simulink model "PilotModelUnitTest"  (R2018b)
settings: Solver=VariableStepAuto  StartTime=0.0  StopTime=100  RelTol=1e-3
values from neighbouring files (symbols this model uses):
  enableHorzMan = 1    [unitTest_PilotModel.m]
  enableVertMan = 0    [unitTest_PilotModel.m]
undefined symbols (not defined in the file or in its folder): ac2dyn_alt0_ft, ac2dyn_con, ac2dyn_lat0_rad, ac2dyn_lon0_rad, daaLogic_turnRate_dps, daaLogic_vertRate_fpm, ddh_ftps2, dh_ftps, dv_ftps2, e_ft, Edot_ftps, h_ft, hdot_ftps, latLonAltState, n_ft, Ndot_ftps, p_radps, phi_rad, phidot_radps, psi_rad, psidot_radps, q_radps, r_radps, theta_rad, thetadot_radps, uasPilot_altitudeK, uasPilot_altitudeOffset, uasPilot_altitudeTheta, uasPilot_coordDelayK, uasPilot_coordDelayMin, uasPilot_coordDelayTheta, uasPilot_desiredTurnRate_dps, uasPilot_desiredVertRate_ftpm, uasPilot_deterministicMode, uasPilot_dt_s, uasPilot_executionDelayMin, uasPilot_executionDelayMu, uasPilot_initialDelayMin, uasPilot_initialDelayMu, uasPilot_maxRelativeHdg, uasPilot_meanUpdateTimes, uasPilot_mentalFilter_climbThresh_fps, uasPilot_mentalFilter_numSamp, uasPilot_mentalFilter_turnThresh_rad, uasPilot_minUpdateTimes, uasPilot_operatorEnabled, uasPilot_probDescend, uasPilot_probFollowMinDev, uasPilot_probLeftTurn, uasPilot_probTurn, uasPilot_reducedClimbAlt_ft, uasPilot_reducedTurnAngle_deg, uasPilot_seedChoose, uasPilot_seedCoordDelay, uasPilot_seedExecutionDelay, uasPilot_seedInitialDelay, uasPilot_seedTurn, uasPilot_seedUpdate, uasPilot_seedVertical, uasPilot_triggerLevel ... (+8)
libraries: simulink x17, NullAircraftEstimateBus x1, uas_pilot_model_r6 x1
(part 1 of 2)
settings Model: Creator=PE29732  LastModifiedBy=BI28030

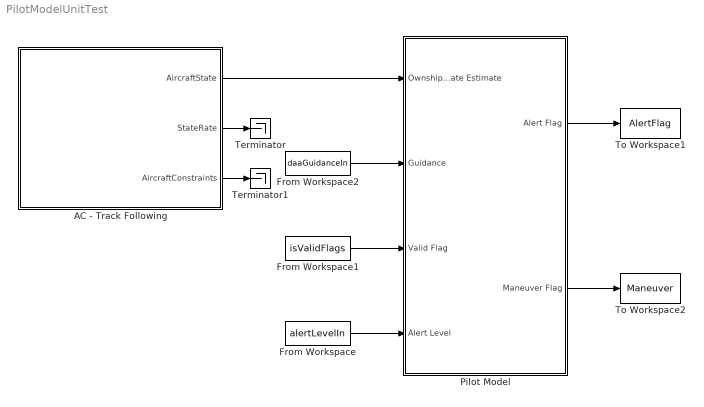
== system PilotModelUnitTest ==
  AC - Track Following : Subsystem  mask(Basic Aircraft Dynamic Model){ts_dynamics=0.1, lat0_rad=ac2dyn_lat0_rad, lon0_rad=ac2dyn_lon0_rad, alt_ft=ac2dyn_alt0_ft, v_ftps_max=ac2dyn_con.maxAirspeed_ftps, v_ftps_min=ac2dyn_con.minAirspeed_ftps, dv_ftpss_max=ac2dyn_con.maxAcceleration_ftpss, dv_ftpss_min=ac2dyn_con.minAcceleration_ftpss, dh_ftps_max=ac2dyn_con.maxVerticalRate_ftps, dh_ftps_min=ac2dyn_con.minVerticalRate_ftps, q_radps_max=ac2dyn_con.maxPitchRate_radps, phi_rad_max=ac2dyn_con.maxBankAngle_rad, dphi_radps_max=ac2dyn_con.maxRollRate_radps, r_radps_max=ac2dyn_con.maxYawRate_radps, pNUM=ac2dyn_con.dynamicsNumeratorRollRate, pDEN=ac2dyn_con.dynamicsDenominatorRollRate, hNUM=ac2dyn_con.dynamicsNumeratorVerticalRate, hDEN=ac2dyn_con.dynamicsDenominatorVerticalRate, rNUM=ac2dyn_con.dynamicsNumeratorYawRate, rDEN=ac2dyn_con.dynamicsDenominatorYawRate}
      mask prompts: ts_dynamics "Dynamics update parameter"; lat0_rad "Latitude of ENU origin (rad)"; lon0_rad "Longitude of ENU origin (rad)"; alt_ft "Height of ENU origin (ft)"; v_ftps_max "Maximum airspeed (ft/s)"; v_ftps_min "Minimum airspeed (ft/s)"; dv_ftpss_max "Maximum acceleration (ft/s/s)"; dv_ftpss_min "Miniimum acceleration (ft/s/s)"; dh_ftps_max "Maximum vertical rate (ft/s)"; dh_ftps_min "Minimum vertical rate (ft/s)"; q_radps_max "Maximum pitch rate (rad/s)"; phi_rad_max "Maximum bank angle (rad)"; dphi_radps_max "Maximum roll rate (rad/s)"; r_radps_max "Maximum yaw rate (rad/s)"; pNUM "Roll rate discrete dynamics numerator (2x1)"; pDEN "Roll rate discrete dynamics denominator (1x1)"; hNUM "Vertical rate discrete dynamics numerator (2x1)"; hDEN "Vertical rate discrete dynamics denominator (1x1)"; rNUM "Yaw rate discrete dynamics numerator (2x1)"; rDEN "Yaw rate discrete dynamics denominator (1x1)"
      mask help:
      | Propagates the aircraft dynamics using 6DOF equations of motion.
      |
      | The class Simple6DOF can be used to programmatically set the parameters of Basic Aircraft Dynamcis blocks.
      mask Help:
      | Propagates the aircraft dynamics using 6DOF equations of motion.
      | 
      | The class Simple6DOF can be used to programmatically set the parameters of Basic Aircraft Dynamcis blocks.
      mask DialogControl ParameterTabVar0 Prompt: Main
      mask DialogControl ParameterTabVar01 Prompt: Constraints
  From Workspace : FromWorkspace  VariableName=alertLevelIn  SampleTime=0
  From Workspace1 : FromWorkspace  VariableName=isValidFlags  SampleTime=0
  From Workspace2 : FromWorkspace  VariableName=daaGuidanceIn  SampleTime=0
  Pilot Model : Subsystem  mask(Heuristic Operator Model){dt=uasPilot_dt_s, operator_enabled=uasPilot_operatorEnabled, deterministicMode=uasPilot_deterministicMode, trigger_level=uasPilot_triggerLevel, mean_initial_delay=uasPilot_initialDelayMu, min_initial_delay=uasPilot_initialDelayMin, coord_delay_k=uasPilot_coordDelayK, coord_delay_theta=uasPilot_coordDelayTheta, coord_delay_min=uasPilot_coordDelayMin, mean_exec_delay=uasPilot_executionDelayMu, min_exec_delay=uasPilot_executionDelayMin, min_upd_times=uasPilot_minUpdateTimes, mean_upd_times=uasPilot_meanUpdateTimes, rng_seed_initial=uasPilot_seedInitialDelay, rng_seed_coord=uasPilot_seedCoordDelay, rng_seed_execution=uasPilot_seedExecutionDelay, rng_seed_update=uasPilot_seedUpdate, prob_follow_min=uasPilot_probFollowMinDev, prob_turn_left=uasPilot_probLeftTurn, prob_descend=uasPilot_probDescend, prob_turn=uasPilot_probTurn, max_hdg_diff=uasPilot_maxRelativeHdg, turn_k=uasPilot_turnK, turn_theta=uasPilot_turnTheta, turn_offset=uasPilot_turnOffset, alt_k=uasPilot_altitudeK, alt_theta=uasPilot_altitudeTheta, alt_offset=uasPilot_altitudeOffset, rng_seed_horz=uasPilot_seedTurn, rng_seed_vert=uasPilot_seedVertical, rng_seed_horz_vs_vert=uasPilot_seedChoose, max_turn_rate=uasPilot_desiredTurnRate_dps, settle_angle=uasPilot_reducedTurnAngle_deg, max_vert_rate=uasPilot_desiredVertRate_ftpm, settle_dist=uasPilot_reducedClimbAlt_ft, mental_filter_samples=uasPilot_mentalFilter_numSamp, mental_filter_turn_thresh=uasPilot_mentalFilter_turnThresh_rad, mental_filter_climb_thresh=uasPilot_mentalFilter_climbThresh_fps, daa_turnRate=daaLogic_turnRate_dps, daa_vertRate=daaLogic_vertRate_fpm}
      mask prompts: dt "Sample Time"; operator_enabled "Enable Pilot Response?"; deterministicMode "Deterministic Mode?"; trigger_level "Trigger Alert Level"; mean_initial_delay "Mean Initial Delay"; min_initial_delay "Minimum Initial Delay"; coord_delay_k "Coordination Delay Shape Parameter (k)"; coord_delay_theta "Coordination Delay Scale Parameter (theta)"; coord_delay_min "Minimum Coordination Delay"; mean_exec_delay "Mean Execution Delay"; min_exec_delay "Minimum Execution Delay"; min_upd_times "Minimum Maneuver Update Times by Alert Level"; mean_upd_times "Mean Maneuver Update Times by Alert Level (sec)"; rng_seed_initial "Random Seed (Initial Delay)"; rng_seed_coord "Random Seed (Coordiantion Delay)"; rng_seed_execution "Random Seed (Execution Delay)"; rng_seed_update "Random Seed (Update Decision)"; prob_follow_min "Probability of Following Minimum Turn"; prob_turn_left "Probability of Turning Left vs. Right"; prob_descend "Probability of Descend vs. CLimb"; prob_turn "Probability of Choosing Turn"; max_hdg_diff "Maximum Heading Difference to Override"; turn_k "Turn Magnitude Shape Parameter (k)"; turn_theta "Turn Magnitude Scale Parameter (theta)"; turn_offset "Turn Magnitude Offset"; alt_k "Altitude Shape Parameter (k)"; alt_theta "Altitude Scale Parameter (theta)"; alt_offset "Altitude Offset"; rng_seed_horz "Random Seed (Horizontal Maneuver Choice)"; rng_seed_vert "Random Seed (Vertical Maneuver Choice)"; rng_seed_horz_vs_vert "Random Seed (Turn vs. Climb)"; max_turn_rate "Desired Turn Rate (deg/s)"; settle_angle "Angle from Desired Heading to Begin Settle (deg)"; max_vert_rate "Desired Vertical Rate (ft/min)"; settle_dist "Distance from Desired Altitude to Begin Settle (ft)"; mental_filter_samples "Number of Samples for Mental Filter"; mental_filter_turn_thresh "Mental Filter Turn Threshold (rad)"; mental_filter_climb_thresh "Mental Filter Climb Threshold (fps)"; daa_turnRate "Max Turn Rate (deg/s)"; daa_vertRate "Max Vertical Rate (fpm)"
      mask help: Identifies pilot response to surveillance estimates of intruder position/course. Either a horizontal or vertical maneuver to maintain well clear.
      mask DialogControl ParameterTabVar0 Prompt: Tab
      mask DialogControl ParameterTabVar01 Prompt: Alert
      mask DialogControl ParameterTabVar012 Prompt: Maneuver Timing
      mask DialogControl ParameterTabVar0123 Prompt: Maneuver Selection
      mask DialogControl ParameterTabVar01234 Prompt: Maneuver Dynamics
      mask DialogControl Container12 Prompt: Pilot Mental Filter
      mask DialogControl Container11 Prompt: DAIDALUS Parameters
  Terminator : Terminator
  Terminator1 : Terminator
  To Workspace1 : ToWorkspace  VariableName=AlertFlag  SaveFormat=Timeseries  SampleTime=-1
  To Workspace2 : ToWorkspace  VariableName=Maneuver  SaveFormat=Timeseries  SampleTime=-1
  wires:
  Pilot Model/1(Alert Flag) -> To Workspace1/1
  Pilot Model/2(Maneuver Flag) -> To Workspace2/1
  AC - Track Following/1(AircraftState) -> Pilot Model/1(Ownship State Estimate)
  AC - Track Following/2(StateRate) -> Terminator/1
  AC - Track Following/3(AircraftConstraints) -> Terminator1/1
  From Workspace/1 -> Pilot Model/4(Alert Level)
  From Workspace1/1 -> Pilot Model/3(Valid Flag)
  From Workspace2/1 -> Pilot Model/2(Guidance)

== system PilotModelUnitTest/AC - Track Following ==
  Follow Trajectory : Subsystem  mask(Follow Trajectory){trajfile=traj_PM.mat}
      mask prompts: trajfile "Trajectory File Name:"
      mask help: Reads trajectory data (North-East-Altitude position and velocity) from specified file. Computes other state variables to follow that trajectory. Ouptuts AircraftState and AircraftStateRate buses.
      mask init:
      | set_param( [ gcb '/Get Trajectory Data/From File' ], 'Filename', trajfile )
  Performance_constraints : Subsystem
  Rate Transition : RateTransition  OutPortSampleTime=0.1
  AircraftState : Outport  OutDataTypeStr=Bus: AircraftState
  StateRate : Outport  Port=2  OutDataTypeStr=Bus: AircraftStateRate
  AircraftConstraints : Outport  Port=3  OutDataTypeStr=Bus: AircraftConstraints
  wires:
  Follow Trajectory/2(State Rate) -> Rate Transition/1
  Follow Trajectory/1(State) -> AircraftState/1
  Performance_constraints/1(AircraftConstraints) -> Follow Trajectory/1(Constraints), AircraftConstraints/1
  Rate Transition/1 -> StateRate/1

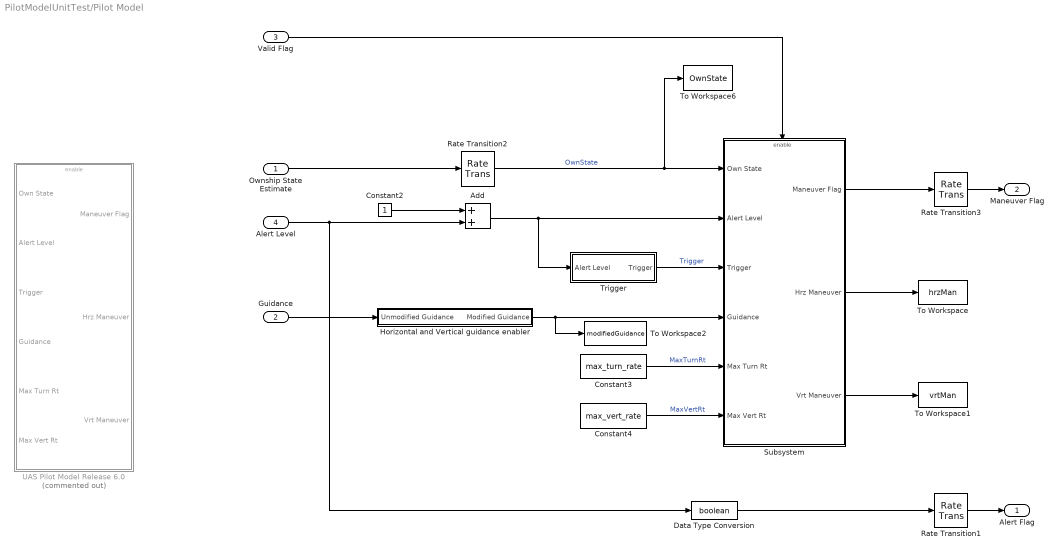
== system PilotModelUnitTest/Pilot Model ==
  Ownship State Estimate : Inport
  Guidance : Inport  Port=2
  Valid Flag : Inport  Port=3
  Alert Level : Inport  Port=4
  Add : Sum
  Constant2 : Constant
  Constant3 : Constant  Value=max_turn_rate
  Constant4 : Constant  Value=max_vert_rate
  Data Type Conversion : DataTypeConversion  OutDataTypeStr=boolean
  Horizontal and Vertical guidance enabler : Subsystem
  Rate Transition1 : RateTransition  OutPortSampleTime=0.1
  Rate Transition2 : RateTransition  OutPortSampleTime=1
  Rate Transition3 : RateTransition  OutPortSampleTime=0.1
  Subsystem : Subsystem
  To Workspace : ToWorkspace  VariableName=hrzMan  SaveFormat=Timeseries  SampleTime=-1
  To Workspace1 : ToWorkspace  VariableName=vrtMan  SaveFormat=Timeseries  SampleTime=-1
  To Workspace2 : ToWorkspace  VariableName=modifiedGuidance  SaveFormat=Timeseries  SampleTime=-1
  To Workspace6 : ToWorkspace  VariableName=OwnState  SaveFormat=Timeseries  SampleTime=-1
  Trigger : Subsystem  mask{trigger_level=trigger_level}
      mask prompts: trigger_level "Alert Level for Trigger"
      mask DialogControl Container6 Prompt: M of N Filter Parameters
      mask DialogControl Container7 Prompt: Hysteresis Parameters
  UAS Pilot Model Release 6.0 : Subsystem  Commented=on  AncestorBlock=CABSAA_ModelLibrary/UAS Pilot Model Release 6.0  TreatAsAtomicUnit=on  mask{dt=uasPilot_dt_s, operator_enabled=uasPilot_operatorEnabled, deterministicMode=uasPilot_deterministicMode, mean_initial_delay=uasPilot_initialDelayMu, min_initial_delay=uasPilot_initialDelayMin, coord_delay_k=uasPilot_coordDelayK, coord_delay_theta=uasPilot_coordDelayTheta, coord_delay_min=uasPilot_coordDelayMin, mean_exec_delay=uasPilot_executionDelayMu, min_exec_delay=uasPilot_executionDelayMin, min_upd_times=uasPilot_minUpdateTimes, mean_upd_times=uasPilot_meanUpdateTimes, rng_seed_initial=uasPilot_seedInitialDelay, rng_seed_coord=uasPilot_seedCoordDelay, rng_seed_execution=uasPilot_seedExecutionDelay, rng_seed_update=uasPilot_seedUpdate, prob_follow_min=uasPilot_probFollowMinDev, prob_turn_left=uasPilot_probLeftTurn, prob_turn_table=uasPilot_probTurn, max_hdg_diff=uasPilot_maxRelativeHdg, prob_descend=uasPilot_probDescend, turn_k=uasPilot_turnK, turn_theta=uasPilot_turnTheta, turn_offset=uasPilot_turnOffset, turn_k_alt=uasPilot_turnK_alt, turn_theta_alt=uasPilot_turnTheta_alt, turn_offset_alt=uasPilot_turnOffset_alt, alt_k=uasPilot_altitudeK, alt_theta=uasPilot_altitudeTheta, alt_offset=uasPilot_altitudeOffset, rng_seed_horz=uasPilot_seedTurn, rng_seed_vert=uasPilot_seedVertical, rng_seed_horz_vs_vert=uasPilot_seedChoose, mental_filter_samples=uasPilot_mentalFilter_numSamp, mental_filter_climb_thresh=uasPilot_mentalFilter_climbThresh_fps, mental_filter_turn_thresh=uasPilot_mentalFilter_turnThresh_rad}
      mask prompts: dt "Sample Time (s)"; operator_enabled "Enable Pilot Model (T/F)"; deterministicMode "Deterministic Mode"; mean_initial_delay "Mean Initial Delay (s)"; min_initial_delay "Minimum Initial Delay (s)"; coord_delay_k "Coordination Delay Gamma Distribution Shape Parameter, k"; coord_delay_theta "Coordination Delay Gamma Distribuition Scale Parameter, theta"; coord_delay_min "Minimum Coordination Delay (s)"; mean_exec_delay "Mean Execution Delay (s)"; min_exec_delay "Minimum Execution Delay (s)"; min_upd_times "Minimum Maneuve Update Times by Alert Level (s)"; mean_upd_times "Mean Maneuver Update Time by Alert Level (s)"; rng_seed_initial "Random Seed (Initial Delay)"; rng_seed_coord "Random Seed (Coord Delay)"; rng_seed_execution "Random Seed (Exec Delay)"; rng_seed_update "Random Seed (Update Delay)"; prob_follow_min "Probability of Following Minimum Guidance"; prob_turn_left "Probability of Turning Left"; prob_turn_table "Probability of Choosing Turn"; max_hdg_diff "Maximum Heading Difference to Override (deg)"; prob_descend "Probability of Descend vs. Climb"; turn_k "Primary Turn Magnitude Gamma Distribution Shape Parameter"; turn_theta "Primary Turn Magnitude Gamma Distribution Scale Parameter"; turn_offset "Primary Turn Magnitude Offset (deg)"; turn_k_alt "Alternate Turn Magnitude Shape Parameter"; turn_theta_alt "Alternate Turn Magnitude Scale Parameter"; turn_offset_alt "Alternate Turn Magnitude Offset"; alt_k "Altitude Gamma Distribution Shape Parameter"; alt_theta "Altitude Gamma Distribution Scale Parameter"; alt_offset "Altitude Offset (ft)"; rng_seed_horz "Random Seed (Horz Maneuver)"; rng_seed_vert "Random Seed (Vert Maneuver)"; rng_seed_horz_vs_vert "Random Seed (Turn vs. Climb)"; mental_filter_samples "Number of Samples for Mental Filter"; mental_filter_climb_thresh "Mental Filter Climb Threshold (fps)"; mental_filter_turn_thresh "Mental Filter Turn Threshold (rad)"
      mask DialogControl DescGroupVar Prompt: UAS Pilot Model
      mask DialogControl DescTextVar Prompt: Response of UAS pilot to intruder causing a DAA alert
  Alert Flag : Outport
  Maneuver Flag : Outport  Port=2
  wires:
  Rate Transition1/1 -> Alert Flag/1
  Ownship State Estimate/1 -> Rate Transition2/1
  Rate Transition3/1 -> Maneuver Flag/1
  Subsystem/1(Maneuver Flag) -> Rate Transition3/1
  Rate Transition2/1 -> To Workspace6/1, Subsystem/1(Own State)  "OwnState"
  Constant2/1 -> Add/1
  Constant3/1 -> Subsystem/5(Max Turn Rt)  "MaxTurnRt"
  Constant4/1 -> Subsystem/6(Max Vert Rt)  "MaxVertRt"
  Data Type Conversion/1 -> Rate Transition1/1
  Trigger/1(Trigger) -> Subsystem/3(Trigger)  "Trigger"
  Valid Flag/1 -> Subsystem/Enable
  Guidance/1 -> Horizontal and Vertical guidance enabler/1(Unmodified Guidance)
  Horizontal and Vertical guidance enabler/1(Modified Guidance) -> Subsystem/4(Guidance), To Workspace2/1
  Alert Level/1 -> Data Type Conversion/1, Add/2
  Add/1 -> Subsystem/2(Alert Level), Trigger/1(Alert Level)
  Subsystem/2(Hrz Maneuver) -> To Workspace/1
  Subsystem/3(Vrt Maneuver) -> To Workspace1/1

== system PilotModelUnitTest/AC - Track Following/Follow Trajectory ==
  Constraints : Inport
  Bus Assignment : BusAssignment  AssignedSignals=p_radps,q_radps,r_radps
  Bus Assignment1 : BusAssignment  AssignedSignals=vdot_fpss,psidot_radps,thetadot_radps,phidot_radps,Ndot_ftps,Edot_ftps,hdot_ftps
  Bus Selector : BusSelector  OutputSignals=dv_ftps2
  Compute Body Rates : Subsystem
  Compute Euler Angles : Subsystem
  Demux : Demux  Outputs=3
  Get Trajectory Data : Subsystem
  Null State Rate : Subsystem
  "Set LLA " : Subsystem  mask{lat0=lat0_rad, lon0=lon0_rad, h0=alt_ft}
      mask prompts: lat0 "ENU latitude origin (rad)"; lon0 "ENU longitude origin (rad)"; h0 "ENU altitude origin (ft)"
  Set State : Subsystem
  Signal Conversion : SignalConversion  OverrideOpt=off
  Signal Conversion1 : SignalConversion  OverrideOpt=off
  State : Outport
  State Rate : Outport  Port=2
  wires:
  Signal Conversion1/1 -> State Rate/1
  Bus Selector/1 -> Bus Assignment1/2  "<dv_ftps2>"
  Compute Euler Angles/3("Phi Dot ") -> Bus Assignment1/5, Compute Body Rates/4(Phi Dot)
  Compute Euler Angles/1(Psi Dot) -> Bus Assignment1/3, Compute Body Rates/2(Psi Dot)
  Demux/3 -> Bus Assignment1/8  "hdot_ftps"
  Null State Rate/1(StateRate) -> Bus Assignment1/1
  Get Trajectory Data/2(xdot) -> Demux/1
  Compute Body Rates/3(r) -> Bus Assignment/4
  Compute Body Rates/2(q) -> Bus Assignment/3
  Compute Body Rates/1(p) -> Bus Assignment/2
  Demux/1 -> Bus Assignment1/6  "Ndot_ftps"
  Demux/2 -> Bus Assignment1/7  "Edot_ftps"
  Compute Euler Angles/2(Theta Dot) -> Bus Assignment1/4, Compute Body Rates/3(Theta Dot)
  Signal Conversion/1 -> State/1
  "Set LLA "/1(State Out) -> Bus Assignment/1
  Bus Assignment/1 -> Signal Conversion/1
  Bus Assignment1/1 -> Signal Conversion1/1
  Set State/1(State) -> Compute Body Rates/1(AircraftState), Compute Euler Angles/1(AircraftState), Bus Selector/1, "Set LLA "/1(State In)
  Constraints/1 -> Compute Euler Angles/2(Constraints)
  Get Trajectory Data/1(x) -> Set State/1(x)

== system PilotModelUnitTest/AC - Track Following/Performance_constraints ==
  Bus Creator : BusCreator  Inputs=16
  Constant : Constant  Value=v_ftps_max
  Constant1 : Constant  Value=v_ftps_min
  Constant10 2x1 : Constant  Value=pNUM
  Constant11 : Constant  Value=pDEN
  Constant12 2x1 : Constant  Value=hNUM
  Constant13 : Constant  Value=hDEN
  Constant14 2x1 : Constant  Value=rNUM
  Constant15 : Constant  Value=rDEN
  Constant2 : Constant  Value=dv_ftpss_max
  Constant3 : Constant  Value=dv_ftpss_min
  Constant4 : Constant  Value=dh_ftps_max
  Constant5 : Constant  Value=dh_ftps_min
  Constant6 : Constant  Value=q_radps_max
  Constant7 : Constant  Value=phi_rad_max
  Constant8 : Constant  Value=dphi_radps_max
  Constant9 : Constant  Value=r_radps_max
  AircraftConstraints : Outport  OutDataTypeStr=Bus: AircraftConstraints
  wires:
  Constant10 2x1/1 -> Bus Creator/11  "pNUM"
  Constant12 2x1/1 -> Bus Creator/13  "hNUM"
  Constant14 2x1/1 -> Bus Creator/15  "rNUM"
  Constant8/1 -> Bus Creator/9  "dphi_radps_max"
  Constant7/1 -> Bus Creator/8  "phi_rad_max"
  Constant6/1 -> Bus Creator/7  "q_radps_max"
  Constant5/1 -> Bus Creator/6  "dh_ftps_min"
  Constant4/1 -> Bus Creator/5  "dh_ftps_max"
  Constant3/1 -> Bus Creator/4  "dv_ftps2_min"
  Constant2/1 -> Bus Creator/3  "dv_ftps2_max"
  Constant1/1 -> Bus Creator/2  "v_ftps_min"
  Constant/1 -> Bus Creator/1  "v_ftps_max"
  Bus Creator/1 -> AircraftConstraints/1
  Constant15/1 -> Bus Creator/16  "rDEN"
  Constant13/1 -> Bus Creator/14  "hDEN"
  Constant11/1 -> Bus Creator/12  "pDEN"
  Constant9/1 -> Bus Creator/10  "r_radps_max"

== system PilotModelUnitTest/Pilot Model/Horizontal and Vertical guidance enabler ==
  Unmodified Guidance : Inport
  " " : Constant  Value=enableVertMan
  " 1" : Constant  Value=enableHorzMan
  Horizontal Band manipulation : MATLAB Function  TreatAsAtomicUnit=on
  Switch : Switch  Criteria=u2 > Threshold
  Switch1 : Switch  Criteria=u2 > Threshold
  Vertical Band manipulation : MATLAB Function  TreatAsAtomicUnit=on
  Modified Guidance : Outport
  wires:
  " "/1 -> Switch/2
  Vertical Band manipulation/1(Guidance_out) -> Switch/3  "Guidance"
  Unmodified Guidance/1 -> Vertical Band manipulation/1(Guidance_in), Switch/1
  " 1"/1 -> Switch1/2
  Switch/1 -> Switch1/1, Horizontal Band manipulation/1(Guidance_in)
  Switch1/1 -> Modified Guidance/1
  Horizontal Band manipulation/1(Guidance_out) -> Switch1/3

== system PilotModelUnitTest/Pilot Model/Subsystem ==
  Own State : Inport
  Alert Level : Inport  Port=2
  Trigger : Inport  Port=3
  Guidance : Inport  Port=4
  Max Turn Rt : Inport  Port=5
  Max Vert Rt : Inport  Port=6
  Enable : EnablePort
  Null AircraftEstimate Bus : NullAircraftEstimateBus/Null AircraftEstimate Bus
  UAS Pilot Model Release 6.1 : uas_pilot_model_r6/UAS Pilot Model Release 6.1  dt=dt  operator_enabled=operator_enabled  deterministicMode=deterministicMode  mean_initial_delay=mean_initial_delay  min_initial_delay=min_initial_delay  coord_delay_k=coord_delay_k  coord_delay_theta=coord_delay_theta  coord_delay_min=coord_delay_min  mean_exec_delay=mean_exec_delay  min_exec_delay=min_exec_delay  min_upd_times=min_upd_times  mean_upd_times=mean_upd_times  rng_seed_initial=rng_seed_initial  rng_seed_coord=rng_seed_coord  rng_seed_execution=rng_seed_execution  rng_seed_update=rng_seed_update  prob_follow_min=prob_follow_min  prob_turn_left=prob_turn_left  prob_turn_table=prob_turn  max_hdg_diff=max_hdg_diff  prob_descend=prob_descend  turn_k=turn_k  turn_theta=turn_theta  turn_offset=turn_offset  turn_k_alt=uasPilot_turnK_alt  turn_theta_alt=uasPilot_turnTheta_alt  turn_offset_alt=uasPilot_turnOffset_alt  alt_k=alt_k  alt_theta=alt_theta  alt_offset=alt_offset  rng_seed_horz=rng_seed_horz  rng_seed_vert=rng_seed_vert  rng_seed_horz_vs_vert=rng_seed_horz_vs_vert  mental_filter_samples=0  mental_filter_climb_thresh=0  mental_filter_turn_thresh=0
  Maneuver Flag : Outport
  Hrz Maneuver : Outport  Port=2
  Vrt Maneuver : Outport  Port=3
  wires:
  UAS Pilot Model Release 6.1/2 -> Hrz Maneuver/1
  UAS Pilot Model Release 6.1/1 -> Maneuver Flag/1
  Alert Level/1 -> UAS Pilot Model Release 6.1/3
  UAS Pilot Model Release 6.1/3 -> Vrt Maneuver/1
  Null AircraftEstimate Bus/1 -> UAS Pilot Model Release 6.1/2
  Max Turn Rt/1 -> UAS Pilot Model Release 6.1/6
  Max Vert Rt/1 -> UAS Pilot Model Release 6.1/7
  Trigger/1 -> UAS Pilot Model Release 6.1/4
  Guidance/1 -> UAS Pilot Model Release 6.1/5
  Own State/1 -> UAS Pilot Model Release 6.1/1

== system PilotModelUnitTest/Pilot Model/Trigger ==
  Alert Level : Inport
  Filter Alerts : Subsystem  AncestorBlock=CABSAA_ModelLibrary/Filter Alerts  mask(Filter Alerts){trigger_level=trigger_level}
      mask prompts: trigger_level "Alert Level for Trigger"
      mask help: Holds alert level for at least the specified time unless the alert level increases.
  Trigger : Outport
  wires:
  Filter Alerts/1(Trigger) -> Trigger/1
  Alert Level/1 -> Filter Alerts/1(Alert Level In)

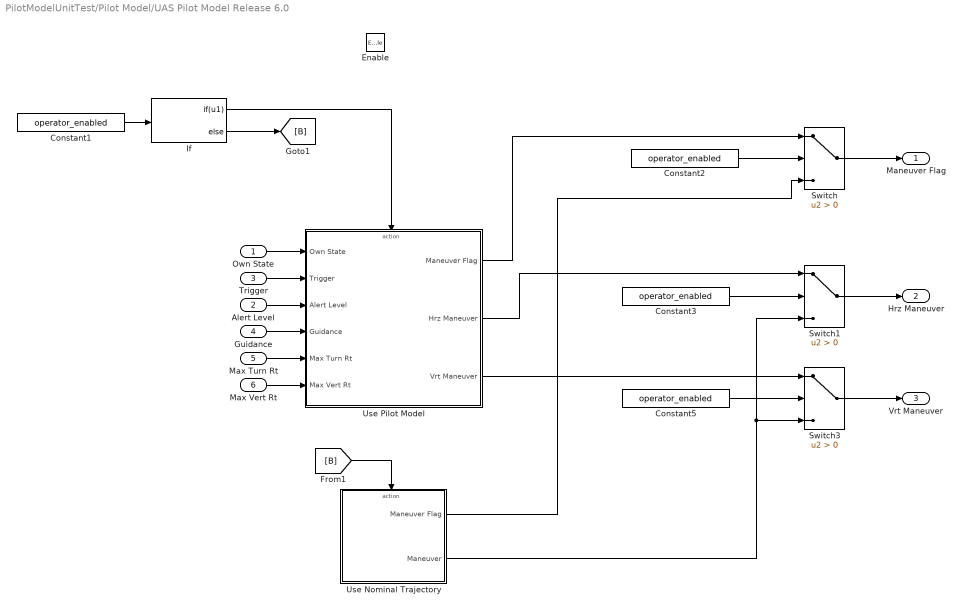
== system PilotModelUnitTest/Pilot Model/UAS Pilot Model Release 6.0 ==
  Own State : Inport  OutDataTypeStr=Bus: AircraftState
  Alert Level : Inport  Port=2
  Trigger : Inport  Port=3
  Guidance : Inport  Port=4
  Max Turn Rt : Inport  Port=5
  Max Vert Rt : Inport  Port=6
  Enable : EnablePort
  Constant{1..3,5} (4 alike) : Constant  Value=operator_enabled  SampleTime=1
  If : If  IfExpression=u1
  Switch : Switch  Criteria=u2 > Threshold
  Switch1 : Switch  Criteria=u2 > Threshold
  Switch3 : Switch  Criteria=u2 > Threshold
  Use Nominal Trajectory : Subsystem  TreatAsAtomicUnit=on
  Use Pilot Model : Subsystem
  Maneuver Flag : Outport  OutDataTypeStr=boolean
  Hrz Maneuver : Outport  Port=2
  Vrt Maneuver : Outport  Port=3
  wires:
  Max Vert Rt/1 -> Use Pilot Model/6(Max Vert Rt)
  Max Turn Rt/1 -> Use Pilot Model/5(Max Turn Rt)
  Alert Level/1 -> Use Pilot Model/3(Alert Level)
  Trigger/1 -> Use Pilot Model/2(Trigger)
  Switch3/1 -> Vrt Maneuver/1
  Switch1/1 -> Hrz Maneuver/1
  Use Nominal Trajectory/2(Maneuver) -> Switch1/3, Switch3/3
  Use Pilot Model/3(Vrt Maneuver) -> Switch3/1
  Constant5/1 -> Switch3/2
  Guidance/1 -> Use Pilot Model/4(Guidance)
  Use Nominal Trajectory/1(Maneuver Flag) -> Switch/3
  Use Pilot Model/2(Hrz Maneuver) -> Switch1/1
  Constant3/1 -> Switch1/2
  Use Pilot Model/1(Maneuver Flag) -> Switch/1
  Constant2/1 -> Switch/2
  Switch/1 -> Maneuver Flag/1
  If/1 -> Use Pilot Model/Action
  Own State/1 -> Use Pilot Model/1(Own State)
  [B] -> Use Nominal Trajectory/Action
  If/2 -> [B]
  Constant1/1 -> If/1

== system PilotModelUnitTest/AC - Track Following/Follow Trajectory/Compute Body Rates ==
  AircraftState : Inport
  Psi Dot : Inport  Port=2
  Theta Dot : Inport  Port=3
  Phi Dot : Inport  Port=4
  Bus Creator : BusCreator  Inputs=3
  Compute p : Subsystem
  Compute q : Subsystem
  Compute r : Subsystem
  p : Outport
  q : Outport  Port=2
  r : Outport  Port=3
  wires:
  Compute r/1(r) -> r/1
  Compute q/1(q) -> q/1
  Compute p/1(p) -> p/1
  Bus Creator/1 -> Compute p/2(Euler Rates), Compute q/2(Euler Rates), Compute r/2(Euler Rates)
  AircraftState/1 -> Compute p/1(State), Compute q/1(State), Compute r/1(State)
  Psi Dot/1 -> Bus Creator/1  "psidot"
  Phi Dot/1 -> Bus Creator/3  "phidot"
  Theta Dot/1 -> Bus Creator/2  "thetadot"

== system PilotModelUnitTest/AC - Track Following/Follow Trajectory/Compute Euler Angles ==
  AircraftState : Inport
  Constraints : Inport  Port=2
  Bus Selector : BusSelector  OutputSignals=psi_rad,theta_rad,phi_rad
  Bus Selector1 : BusSelector  OutputSignals=dphi_radps_max
  Discrete Derivative : simulink/Discrete/Discrete Derivative  gainval=1.0  ICPrevScaledInput=0.0  OutMin=[]  OutMax=[]  OutDataType=fixdt(1, 16)  OutScaling=2^-10  DoSatur=off
  Discrete Derivative1 : simulink/Discrete/Discrete Derivative  gainval=1.0  ICPrevScaledInput=0.0  OutMin=[]  OutMax=[]  OutDataType=fixdt(1, 16)  OutScaling=2^-10  DoSatur=off
  Discrete Derivative2 : simulink/Discrete/Discrete Derivative  gainval=1.0  ICPrevScaledInput=0.0  OutMin=[]  OutMax=[]  OutDataType=fixdt(1, 16)  OutScaling=2^-10  DoSatur=off
  IC : InitialCondition  Value=0
  IC1 : InitialCondition  Value=0
  IC2 : InitialCondition  Value=0
  Saturation Dynamic : simulink/Discontinuities/Saturation Dynamic  OutMin=[]  OutMax=[]  OutDataTypeStr=Inherit: Same as second input  OutDataType=fixdt(1, 16)  OutScaling=2^-10  DoSatur=off
  Unary Minus : UnaryMinus
  Psi Dot : Outport
  Theta Dot : Outport  Port=2
  "Phi Dot " : Outport  Port=3
  wires:
  Constraints/1 -> Bus Selector1/1
  IC2/1 -> Saturation Dynamic/2
  IC1/1 -> Theta Dot/1
  IC/1 -> Psi Dot/1
  Discrete Derivative2/1 -> IC2/1
  Discrete Derivative1/1 -> IC1/1
  Discrete Derivative/1 -> IC/1
  Bus Selector/3 -> Discrete Derivative2/1  "<phi_rad>"
  Bus Selector/2 -> Discrete Derivative1/1  "<theta_rad>"
  Bus Selector/1 -> Discrete Derivative/1  "<psi_rad>"
  AircraftState/1 -> Bus Selector/1
  Saturation Dynamic/1 -> "Phi Dot "/1
  Bus Selector1/1 -> Unary Minus/1, Saturation Dynamic/1  "<dphi_radps_max>"
  Unary Minus/1 -> Saturation Dynamic/3

== system PilotModelUnitTest/AC - Track Following/Follow Trajectory/Get Trajectory Data ==
  Compute Accel : Subsystem
  Compute Accel1 : Subsystem
  Compute Bank Angle : Subsystem
  Demux : Demux  Outputs=6
  Divide : Product  Inputs=*/
  From File : FromFile  FileName=traj_PM.mat  SampleTime=0.1
  Math Function : Math  Operator=square  SaturateOnIntegerOverflow=on
  Mux : Mux  Inputs=3
  Mux1 : Mux  Inputs=10
  Mux2 : Mux  Inputs=3
  Sqrt : Sqrt  SaturateOnIntegerOverflow=on
  Sum of Elements : Sum  Inputs=+
  To Workspace : ToWorkspace  VariableName=traj1  SaveFormat=Timeseries  SampleTime=-1
  Trigonometric Function : Trigonometry  Operator=asin
  Trigonometric Function1 : Trigonometry  Operator=atan2
  x : Outport
  xdot : Outport  Port=2
  wires:
  Mux/1 -> xdot/1
  Compute Accel1/1(accel) -> Mux1/10  "hdd"
  Demux/5 -> Mux2/2, Trigonometric Function1/1, Mux/2
  Divide/1 -> Trigonometric Function/1
  Trigonometric Function1/1 -> Mux1/5, Compute Bank Angle/2(psi)  "psi"
  Trigonometric Function/1 -> Mux1/6  "theta"
  Compute Bank Angle/1(phi) -> Mux1/7  "phi"
  Compute Accel/1(accel) -> Mux1/8  "a"
  Mux1/1 -> x/1
  Sqrt/1 -> Divide/2, Mux1/1, Compute Bank Angle/1(speed), Compute Accel/1(speed)  "speed"
  Sum of Elements/1 -> Sqrt/1
  Math Function/1 -> Sum of Elements/1
  Mux2/1 -> Math Function/1
  Demux/6 -> Mux1/9, Compute Accel1/1(speed), Divide/1, Mux2/3, Mux/3  "hdot"
  Demux/4 -> Mux2/1, Trigonometric Function1/2, Mux/1
  Demux/3 -> Mux1/4  "Alt"
  Demux/2 -> Mux1/3  "E"
  Demux/1 -> Mux1/2  "N"
  From File/1 -> To Workspace/1, Demux/1

== system PilotModelUnitTest/AC - Track Following/Follow Trajectory/Null State Rate ==
  Bus Creator : BusCreator  Inputs='vdot_fpss','Ndot_ftps','Edot_ftps','hdot_ftps','psidot_radps','thetadot_radps','phidot_radps'  OutDataTypeStr=Bus: AircraftStateRate
  Constant{,1..6} (7 alike) : Constant  Value=0
  StateRate : Outport  OutDataTypeStr=Bus: AircraftStateRate
  wires:
  Constant6/1 -> Bus Creator/7  "phidot_radps"
  Constant5/1 -> Bus Creator/6  "thetadot_radps"
  Constant4/1 -> Bus Creator/5  "psidot_radps"
  Constant3/1 -> Bus Creator/4  "hdot_ftps"
  Constant2/1 -> Bus Creator/3  "Edot_ftps"
  Constant1/1 -> Bus Creator/2  "Ndot_ftps"
  Constant/1 -> Bus Creator/1  "vdot_fpss"
  Bus Creator/1 -> StateRate/1

== system PilotModelUnitTest/AC - Track Following/Follow Trajectory/Set LLA  ==
  State In : Inport
  Bus Assignment : BusAssignment  AssignedSignals=latLonAltState.lat_rad,latLonAltState.lon_rad,latLonAltState.dlat_radps,latLonAltState.dlon_radps,latLonAltState.alt_ft,latLonAltState.dalt_ftps
  Bus Selector : BusSelector  OutputSignals=e_ft,n_ft,h_ft,v_ftps,psi_rad,theta_rad
  Constant : Constant  Value=lat0
  Constant7 : Constant  Value=lon0
  Constant8 : Constant  Value=h0
  MATLAB Function : MATLAB Function  TreatAsAtomicUnit=on
  State Out : Outport
  wires:
  Bus Selector/6 -> MATLAB Function/6(theta_rad)  "<theta_rad>"
  Bus Selector/5 -> MATLAB Function/5(psi_rad)  "<psi_rad>"
  Bus Selector/4 -> MATLAB Function/4(v_ftps)  "<v_ftps>"
  Bus Selector/3 -> MATLAB Function/3(u_ft)  "<h_ft>"
  Bus Selector/2 -> MATLAB Function/2(n_ft)  "<n_ft>"
  Bus Selector/1 -> MATLAB Function/1(e_ft)  "<e_ft>"
  Constant8/1 -> MATLAB Function/9(h0)
  Constant7/1 -> MATLAB Function/8(lon0)
  Constant/1 -> MATLAB Function/7(lat0)
  State In/1 -> Bus Selector/1, Bus Assignment/1
  Bus Assignment/1 -> State Out/1
  MATLAB Function/6(dalt_ftps) -> Bus Assignment/7  "dalt_ftps"
  MATLAB Function/5(alt_ft) -> Bus Assignment/6  "alt_ft"
  MATLAB Function/4(dlon_radps) -> Bus Assignment/5  "dlon_radps"
  MATLAB Function/3(dlat_radps) -> Bus Assignment/4  "dlat_radps"
  MATLAB Function/2(lon_rad) -> Bus Assignment/3  "lon_rad"
  MATLAB Function/1(lat_rad) -> Bus Assignment/2  "lat_rad"

== system PilotModelUnitTest/AC - Track Following/Follow Trajectory/Set State ==
  x : Inport
  Bus Assignment : BusAssignment  AssignedSignals=v_ftps,n_ft,e_ft,h_ft,psi_rad,theta_rad,phi_rad,dv_ftps2,dh_ftps,ddh_ftps2
  Demux : Demux  Outputs=10
  Null AircraftState : Subsystem
  State : Outport
  wires:
  Demux/10 -> Bus Assignment/11
  Demux/9 -> Bus Assignment/10
  Bus Assignment/1 -> State/1
  Null AircraftState/1(State) -> Bus Assignment/1
  Demux/7 -> Bus Assignment/8  "phi"
  x/1 -> Demux/1
  Demux/6 -> Bus Assignment/7  "theta"
  Demux/5 -> Bus Assignment/6  "psi"
  Demux/4 -> Bus Assignment/5  "h"
  Demux/3 -> Bus Assignment/4  "E"
  Demux/2 -> Bus Assignment/3  "N"
  Demux/1 -> Bus Assignment/2  "v"
  Demux/8 -> Bus Assignment/9  "a"

== system PilotModelUnitTest/Pilot Model/Trigger/Filter Alerts ==
  Alert Level In : Inport
  Constant6 : Constant  Value=trigger_level
  Relational Operator : RelationalOperator  OutDataTypeStr=boolean  RndMeth=Nearest
  To Workspace : ToWorkspace  VariableName=AlertLevelToCompare  SaveFormat=Timeseries  SampleTime=-1
  Trigger : Outport
  wires:
  Relational Operator/1 -> Trigger/1
  Constant6/1 -> Relational Operator/2
  Alert Level In/1 -> To Workspace/1, Relational Operator/1

== system PilotModelUnitTest/Pilot Model/UAS Pilot Model Release 6.0/Use Nominal Trajectory ==
  Action Port : ActionPort  ActionType=else
  Constant : Constant  Value=false
  Null Maneuver : Subsystem
  Maneuver Flag : Outport  InitialOutput=0
  Maneuver : Outport  Port=2  InitialOutput=0
  wires:
  Constant/1 -> Maneuver Flag/1
  Null Maneuver/1(Null) -> Maneuver/1

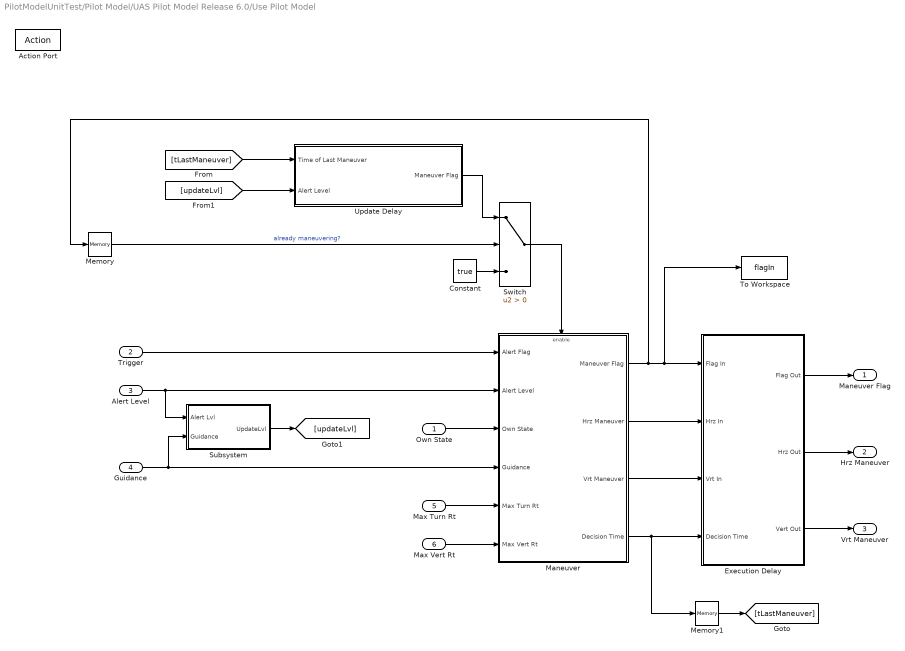
== system PilotModelUnitTest/Pilot Model/UAS Pilot Model Release 6.0/Use Pilot Model ==
  Own State : Inport  OutDataTypeStr=Bus: AircraftState
  Trigger : Inport  Port=2
  Alert Level : Inport  Port=3
  Guidance : Inport  Port=4
  Max Turn Rt : Inport  Port=5
  Max Vert Rt : Inport  Port=6
  Action Port : ActionPort  ActionType=then
  Constant : Constant  Value=true
  Execution Delay : Subsystem
  Maneuver : Subsystem
  Memory : Memory  InheritSampleTime=on
  Memory1 : Memory  InheritSampleTime=on
  Subsystem : Subsystem
  Switch : Switch  Criteria=u2 > Threshold
  To Workspace : ToWorkspace  VariableName=flagIn  SaveFormat=Timeseries  SampleTime=-1
  Update Delay : Subsystem
  Maneuver Flag : Outport  OutDataTypeStr=boolean
  Hrz Maneuver : Outport  Port=2
  Vrt Maneuver : Outport  Port=3
  wires:
  Execution Delay/3(Vert Out) -> Vrt Maneuver/1
  Execution Delay/2(Hrz Out) -> Hrz Maneuver/1
  Execution Delay/1(Flag Out) -> Maneuver Flag/1
  Max Vert Rt/1 -> Maneuver/6(Max Vert Rt)
  Max Turn Rt/1 -> Maneuver/5(Max Turn Rt)
  [updateLvl] -> Update Delay/2(Alert Level)
  Subsystem/1(UpdateLvl) -> [updateLvl]
  [tLastManeuver] -> Update Delay/1(Time of Last Maneuver)
  Memory1/1 -> [tLastManeuver]
  Maneuver/4(Decision Time) -> Execution Delay/4(Decision Time), Memory1/1
  Update Delay/1(Maneuver Flag) -> Switch/1
  Maneuver/3(Vrt Maneuver) -> Execution Delay/3(Vrt In)
  Maneuver/2(Hrz Maneuver) -> Execution Delay/2(Hrz In)
  Switch/1 -> Maneuver/Enable
  Alert Level/1 -> Maneuver/2(Alert Level), Subsystem/1(Alert Lvl)
  Trigger/1 -> Maneuver/1(Alert Flag)
  Own State/1 -> Maneuver/3(Own State)
  Memory/1 -> Switch/2  "already maneuvering?"
  Constant/1 -> Switch/3
  Guidance/1 -> Maneuver/4(Guidance), Subsystem/2(Guidance)
  Maneuver/1(Maneuver Flag) -> Memory/1, To Workspace/1, Execution Delay/1(Flag In)

== system PilotModelUnitTest/AC - Track Following/Follow Trajectory/Compute Body Rates/Compute p ==
  State : Inport
  Euler Rates : Inport  Port=2
  Add : Sum
  Bus Selector : BusSelector  OutputSignals=theta_rad
  Bus Selector1 : BusSelector  OutputSignals=psidot,phidot
  Product : Product
  Trigonometric Function : Trigonometry
  Unary Minus : UnaryMinus
  p : Outport
  wires:
  Add/1 -> p/1
  Unary Minus/1 -> Product/1
  Bus Selector1/2 -> Add/2  "<phidot>"
  Product/1 -> Add/1
  Trigonometric Function/1 -> Unary Minus/1
  State/1 -> Bus Selector/1
  Euler Rates/1 -> Bus Selector1/1
  Bus Selector/1 -> Trigonometric Function/1  "<theta_rad>"
  Bus Selector1/1 -> Product/2  "<psidot>"

== system PilotModelUnitTest/AC - Track Following/Follow Trajectory/Compute Body Rates/Compute q ==
  State : Inport
  Euler Rates : Inport  Port=2
  Add : Sum
  Bus Selector : BusSelector  OutputSignals=phi_rad,theta_rad
  Bus Selector1 : BusSelector  OutputSignals=thetadot,psidot
  Product : Product
  Product1 : Product  Inputs=3
  Trigonometric Function : Trigonometry  Operator=cos
  Trigonometric Function1 : Trigonometry  Operator=cos
  Trigonometric Function2 : Trigonometry
  q : Outport
  wires:
  Add/1 -> q/1
  Product1/1 -> Add/2
  Bus Selector1/2 -> Product1/3  "<psidot>"
  Trigonometric Function1/1 -> Product1/2
  Trigonometric Function2/1 -> Product1/1
  Bus Selector/2 -> Trigonometric Function1/1  "<theta_rad>"
  Bus Selector1/1 -> Product/2  "<thetadot>"
  Bus Selector/1 -> Trigonometric Function/1, Trigonometric Function2/1  "<phi_rad>"
  Trigonometric Function/1 -> Product/1
  Product/1 -> Add/1
  State/1 -> Bus Selector/1
  Euler Rates/1 -> Bus Selector1/1

== system PilotModelUnitTest/AC - Track Following/Follow Trajectory/Compute Body Rates/Compute r ==
  State : Inport
  Euler Rates : Inport  Port=2
  Add : Sum
  Bus Selector : BusSelector  OutputSignals=phi_rad,theta_rad
  Bus Selector1 : BusSelector  OutputSignals=thetadot,psidot
  Product : Product
  Product1 : Product  Inputs=3
  Trigonometric Function : Trigonometry
  Trigonometric Function1 : Trigonometry  Operator=cos
  Trigonometric Function2 : Trigonometry  Operator=cos
  Unary Minus : UnaryMinus
  r : Outport
  wires:
  Unary Minus/1 -> Product/1
  Add/1 -> r/1
  Product1/1 -> Add/2
  Bus Selector1/2 -> Product1/3  "<psidot>"
  Trigonometric Function1/1 -> Product1/2
  Trigonometric Function2/1 -> Product1/1
  Bus Selector/2 -> Trigonometric Function1/1  "<theta_rad>"
  Bus Selector1/1 -> Product/2  "<thetadot>"
  Bus Selector/1 -> Trigonometric Function/1, Trigonometric Function2/1  "<phi_rad>"
  Trigonometric Function/1 -> Unary Minus/1
  Product/1 -> Add/1
  State/1 -> Bus Selector/1
  Euler Rates/1 -> Bus Selector1/1

== system PilotModelUnitTest/AC - Track Following/Follow Trajectory/Get Trajectory Data/Compute Accel ==
  speed : Inport
  Discrete Derivative : simulink/Discrete/Discrete Derivative  gainval=1.0  ICPrevScaledInput=0.0  OutMin=[]  OutMax=[]  OutDataType=fixdt(1, 16)  OutScaling=2^-10  DoSatur=off
  accel : Outport
  wires:
  Discrete Derivative/1 -> accel/1
  speed/1 -> Discrete Derivative/1

== system PilotModelUnitTest/AC - Track Following/Follow Trajectory/Get Trajectory Data/Compute Accel1 ==
  speed : Inport
  Discrete Derivative : simulink/Discrete/Discrete Derivative  gainval=1.0  ICPrevScaledInput=0.0  OutMin=[]  OutMax=[]  OutDataType=fixdt(1, 16)  OutScaling=2^-10  DoSatur=off
  accel : Outport
  wires:
  Discrete Derivative/1 -> accel/1
  speed/1 -> Discrete Derivative/1

== system PilotModelUnitTest/AC - Track Following/Follow Trajectory/Get Trajectory Data/Compute Bank Angle ==
  speed : Inport
  psi : Inport  Port=2
  Constant : Constant  Value=32.2
  Discrete Derivative : simulink/Discrete/Discrete Derivative  gainval=1.0  ICPrevScaledInput=0.0  OutMin=[]  OutMax=[]  OutDataType=fixdt(1, 16)  OutScaling=2^-10  DoSatur=off
  Divide : Product  Inputs=*/
  IC : InitialCondition  Value=0
  Product : Product
  Trigonometric Function : Trigonometry  Operator=atan
  phi : Outport
  wires:
  IC/1 -> Product/2
  Trigonometric Function/1 -> phi/1
  Divide/1 -> Trigonometric Function/1
  Constant/1 -> Divide/2
  Product/1 -> Divide/1
  psi/1 -> Discrete Derivative/1  "psi"
  speed/1 -> Product/1  "speed"
  Discrete Derivative/1 -> IC/1  "psidot"

== system PilotModelUnitTest/AC - Track Following/Follow Trajectory/Set State/Null AircraftState ==
  Bus Creator : BusCreator  Inputs='latLonAltState','v_ftps','n_ft','e_ft','h_ft','psi_rad','theta_rad','phi_rad','p_radps','q_radps','r_radps','dv_ftps2','dh_ftps','ddh_ftps2'  OutDataTypeStr=Bus: AircraftState
  Constant{,1..12} (13 alike) : Constant  Value=0
  Null LatLonAltMeasurement : Subsystem
  State : Outport
  wires:
  Null LatLonAltMeasurement/1(LLA) -> Bus Creator/1  "latLonAltState"
  Constant/1 -> Bus Creator/2  "v_ftps"
  Constant12/1 -> Bus Creator/14  "ddh_ftps2"
  Constant1/1 -> Bus Creator/3  "n_ft"
  Bus Creator/1 -> State/1
  Constant6/1 -> Bus Creator/8  "phi_rad"
  Constant10/1 -> Bus Creator/12  "dv_ftps2"
  Constant7/1 -> Bus Creator/9  "p_radps"
  Constant5/1 -> Bus Creator/7  "theta_rad"
  Constant4/1 -> Bus Creator/6  "psi_rad"
  Constant8/1 -> Bus Creator/10  "q_radps"
  Constant9/1 -> Bus Creator/11  "r_radps"
  Constant3/1 -> Bus Creator/5  "h_ft"
  Constant2/1 -> Bus Creator/4  "e_ft"
  Constant11/1 -> Bus Creator/13  "dh_ftps"

== system PilotModelUnitTest/Pilot Model/UAS Pilot Model Release 6.0/Use Nominal Trajectory/Null Maneuver ==
  Bus Creator : BusCreator  Inputs=5  OutDataTypeStr=Bus: AvoidanceManeuver
  Constant{,1..3} (4 alike) : Constant  Value=0
  Digital Clock : DigitalClock  SampleTime=dt
  Null : Outport
  wires:
  Constant3/1 -> Bus Creator/4  "reference_state"
  Bus Creator/1 -> Null/1
  Digital Clock/1 -> Bus Creator/1  "time"
  Constant1/1 -> Bus Creator/3  "desired_state"
  Constant/1 -> Bus Creator/2  "type"
  Constant2/1 -> Bus Creator/5  "wc_flag"

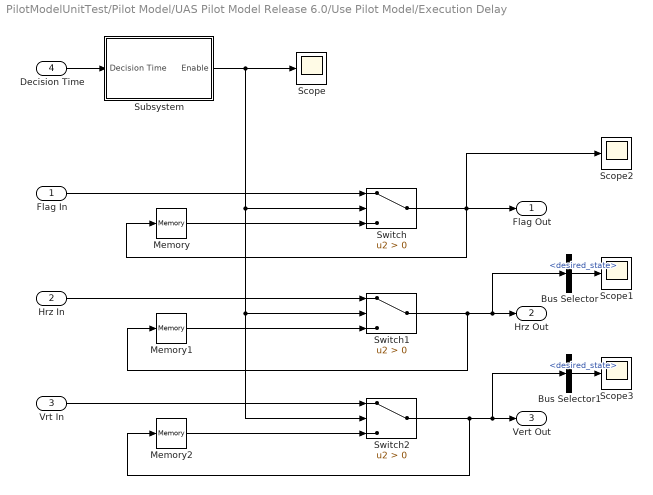
== system PilotModelUnitTest/Pilot Model/UAS Pilot Model Release 6.0/Use Pilot Model/Execution Delay ==
  Flag In : Inport
  Hrz In : Inport  Port=2
  Vrt In : Inport  Port=3
  Decision Time : Inport  Port=4
  Bus Selector : BusSelector  OutputSignals=desired_state
  Bus Selector1 : BusSelector  OutputSignals=desired_state
  Memory : Memory  InheritSampleTime=on
  Memory1 : Memory  InheritSampleTime=on
  Memory2 : Memory  InheritSampleTime=on
  Scope{,1..3} (4 alike) : Scope
  Subsystem : Subsystem
  Switch : Switch  Criteria=u2 > Threshold
  Switch1 : Switch  Criteria=u2 > Threshold
  Switch2 : Switch  Criteria=u2 > Threshold
  Flag Out : Outport
  Hrz Out : Outport  Port=2
  Vert Out : Outport  Port=3
  wires:
  Bus Selector1/1 -> Scope3/1  "<desired_state>"
  Switch2/1 -> Vert Out/1, Bus Selector1/1, Memory2/1
  Bus Selector/1 -> Scope1/1  "<desired_state>"
  Decision Time/1 -> Subsystem/1(Decision Time)
  Subsystem/1(Enable) -> Switch2/2, Switch1/2, Switch/2, Scope/1
  Memory2/1 -> Switch2/3
  Memory1/1 -> Switch1/3
  Memory/1 -> Switch/3
  Hrz In/1 -> Switch1/1
  Vrt In/1 -> Switch2/1
  Flag In/1 -> Switch/1
  Switch1/1 -> Hrz Out/1, Bus Selector/1, Memory1/1
  Switch/1 -> Flag Out/1, Memory/1, Scope2/1

== system PilotModelUnitTest/Pilot Model/UAS Pilot Model Release 6.0/Use Pilot Model/Maneuver ==
  Alert Flag : Inport
  Alert Level : Inport  Port=2
  Own State : Inport  Port=3
  Guidance : Inport  Port=4
  Max Turn Rt : Inport  Port=5
  Max Vert Rt : Inport  Port=6
  Enable : EnablePort
  Coordination Delay : Subsystem
  Initial Delay : Subsystem
  Logical Operator : Logic  Operator=OR  AllPortsSameDT=off  OutDataTypeStr=boolean
  Maneuver Selection : Subsystem  TreatAsAtomicUnit=on
  Memory : Memory  InheritSampleTime=on
  Scope1 : Scope
  Maneuver Flag : Outport
  Hrz Maneuver : Outport  Port=2
  Vrt Maneuver : Outport  Port=3
  Decision Time : Outport  Port=4
  wires:
  Maneuver Selection/1(Maneuver Flag) -> Memory/1, Maneuver Flag/1
  Maneuver Selection/2(Hrz Maneuver) -> Hrz Maneuver/1
  Maneuver Selection/3(Vrt Maneuver) -> Vrt Maneuver/1
  Maneuver Selection/4(Decision Time) -> Decision Time/1
  Max Vert Rt/1 -> Maneuver Selection/4(Max Vert Rt)
  Max Turn Rt/1 -> Maneuver Selection/3(Max Turn Rt)
  Logical Operator/1 -> Initial Delay/2(Alert Flag), Coordination Delay/3(Alert Flag)
  Alert Flag/1 -> Logical Operator/2
  Own State/1 -> Maneuver Selection/1(Own State)
  Coordination Delay/1(Flag Out) -> Scope1/1, Maneuver Selection/Enable
  Alert Level/1 -> Coordination Delay/4(Alert Level)
  Initial Delay/1(Flag Out) -> Coordination Delay/2(Flag In)
  Memory/1 -> Initial Delay/1(Maneuver Flag), Logical Operator/1, Coordination Delay/1(Maneuver Flag)
  Guidance/1 -> Maneuver Selection/2(Guidance)

== system PilotModelUnitTest/Pilot Model/UAS Pilot Model Release 6.0/Use Pilot Model/Subsystem ==
  note: Alert Levels:
      | 0 = no alert
      | 1 = proximate alert
      | 2 = preventive alert
      | 3 = corrective alert
      | 4 = warning alert
      | 5 = recovery bands or WCV
  note: See if horizontal guidance includes any recovery bands (value =1)
  note: Pass through current alert level unless any recovery guidance is present, in which case set alert level to 5
  Alert Lvl : Inport
  Guidance : Inport  Port=2
  Compare To Constant : simulink/Logic and Bit Operations/Compare To Constant  relop===  const=1  OutDataTypeStr=boolean
  Compare To Zero : simulink/Logic and Bit Operations/Compare To Zero  relop=>  OutDataTypeStr=boolean
  Constant : Constant  Value=5
  Selector : Selector  InputPortWidth=283  IndexOptions=Index vector (dialog)  Indices=[1:271]  OutputSizes=1
  Sum of Elements : Sum  Inputs=+
  Switch1 : Switch  Criteria=u2 > Threshold
  UpdateLvl : Outport
  wires:
  Selector/1 -> Compare To Constant/1
  Sum of Elements/1 -> Compare To Zero/1
  Compare To Constant/1 -> Sum of Elements/1
  Guidance/1 -> Selector/1
  Alert Lvl/1 -> Switch1/3
  Constant/1 -> Switch1/1
  Compare To Zero/1 -> Switch1/2
  Switch1/1 -> UpdateLvl/1

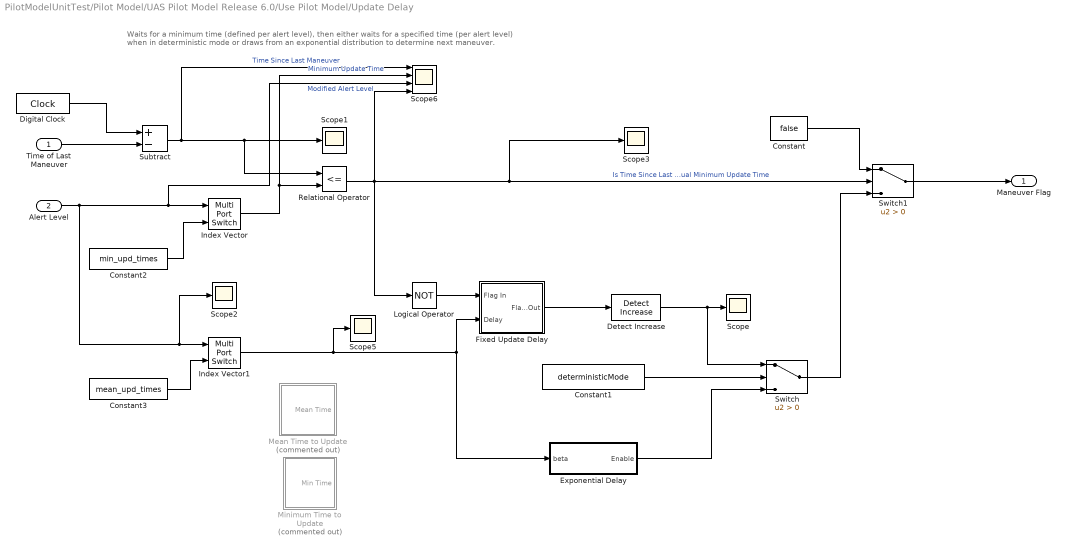
== system PilotModelUnitTest/Pilot Model/UAS Pilot Model Release 6.0/Use Pilot Model/Update Delay ==
  note: Waits for a minimum time (defined per alert level), then either waits for a specified time (per alert level)
      | when in deterministic mode or draws from an exponential distribution to determine next maneuver.
  Time of Last Maneuver : Inport
  Alert Level : Inport  Port=2
  Constant : Constant  Value=false
  Constant1 : Constant  Value=deterministicMode
  Constant2 : Constant  Value=min_upd_times
  Constant3 : Constant  Value=mean_upd_times
  Detect Increase : simulink/Logic and Bit Operations/Detect Increase  vinit=0.0  OutDataTypeStr=boolean
  Digital Clock : DigitalClock
  Exponential Delay : Subsystem  mask(Exponentially-Distributed Delay){dt=dt, seed=rng_seed_update}
      mask prompts: dt "Sample time (seconds):"; seed "Random seed:"
      mask help:
      | Outputs whether a delay follows an exponential distribution with the specified mean time has completed.
      |
      | Because the exponential distribution is memoryless, the probability of finishing the delay at the current timestep is independent of previous timesteps.
  Fixed Update Delay : Subsystem
  Index Vector : MultiPortSwitch  DataPortOrder=Zero-based contiguous  Inputs=1  zeroidx=on
  Index Vector1 : MultiPortSwitch  DataPortOrder=Zero-based contiguous  Inputs=1  zeroidx=on
  Logical Operator : Logic  Operator=NOT  AllPortsSameDT=off  OutDataTypeStr=boolean
  Mean Time to Update : Subsystem  Commented=on
  Minimum Time to Update : Subsystem  Commented=on
  Relational Operator : RelationalOperator  Operator=<=  OutDataTypeStr=boolean  RndMeth=Nearest
  Scope{,1..3,5} (5 alike) : Scope
  Scope6 : Scope  NumInputPorts=4
  Subtract : Sum  Inputs=+-
  Switch : Switch  Criteria=u2 > Threshold
  Switch1 : Switch  Criteria=u2 > Threshold
  Maneuver Flag : Outport
  wires:
  Subtract/1 -> Relational Operator/1, Scope1/1, Scope6/1  "Time Since Last Maneuver"
  Digital Clock/1 -> Subtract/1
  Time of Last Maneuver/1 -> Subtract/2
  Switch/1 -> Switch1/3
  Index Vector1/1 -> Scope5/1, Fixed Update Delay/2(Delay), Exponential Delay/1(beta)
  Constant/1 -> Switch1/1
  Index Vector/1 -> Scope6/2, Relational Operator/2  "Minimum Update Time"
  Constant3/1 -> Index Vector1/2
  Constant2/1 -> Index Vector/2
  Alert Level/1 -> Scope6/3, Index Vector/1, Scope2/1, Index Vector1/1  "Modified Alert Level"
  Detect Increase/1 -> Switch/1, Scope/1
  Fixed Update Delay/1(Flag Out) -> Detect Increase/1
  Relational Operator/1 -> Scope6/4, Logical Operator/1, Scope3/1, Switch1/2  "Is Time Since Last Maneuver Less than or equal Minimum Update Time"
  Exponential Delay/1(Enable) -> Switch/3
  Constant1/1 -> Switch/2
  Switch1/1 -> Maneuver Flag/1
  Logical Operator/1 -> Fixed Update Delay/1(Flag In)

== system PilotModelUnitTest/AC - Track Following/Follow Trajectory/Set State/Null AircraftState/Null LatLonAltMeasurement ==
  Bus Creator : BusCreator  Inputs='lat_rad','lon_rad','dlat_radps','dlon_radps','alt_ft','dalt_ftps'  OutDataTypeStr=Bus: LatLonAltMeasurement
  Constant{,1..5} (6 alike) : Constant  Value=0
  LLA : Outport
  wires:
  Constant1/1 -> Bus Creator/2  "lon_rad"
  Bus Creator/1 -> LLA/1
  Constant4/1 -> Bus Creator/5  "alt_ft"
  Constant5/1 -> Bus Creator/6  "dalt_ftps"
  Constant3/1 -> Bus Creator/4  "dlon_radps"
  Constant/1 -> Bus Creator/1  "lat_rad"
  Constant2/1 -> Bus Creator/3  "dlat_radps"

== system PilotModelUnitTest/Pilot Model/UAS Pilot Model Release 6.0/Use Pilot Model/Execution Delay/Subsystem ==
  Decision Time : Inport
  Compare To Zero : simulink/Logic and Bit Operations/Compare To Zero  relop===  OutDataTypeStr=boolean
  Constant : Constant  Value=mean_exec_delay
  Constant1 : Constant  Value=deterministicMode
  Constant2 : Constant  Value=false
  Constant3 : Constant  Value=min_exec_delay
  Detect Increase : simulink/Logic and Bit Operations/Detect Increase  vinit=0.0  OutDataTypeStr=boolean
  Digital Clock : DigitalClock
  Exponential Delay : Subsystem  mask(Exponentially-Distributed Delay){dt=dt, seed=rng_seed_execution}
      mask prompts: dt "Sample time (seconds):"; seed "Random seed:"
      mask help:
      | Outputs whether a delay follows an exponential distribution with the specified mean time has completed.
      |
      | Because the exponential distribution is memoryless, the probability of finishing the delay at the current timestep is independent of previous timesteps.
  Fixed Update Delay : Subsystem
  Logical Operator : Logic  Operator=NOT  AllPortsSameDT=off  OutDataTypeStr=boolean
  Logical Operator1 : Logic  Operator=OR  AllPortsSameDT=off  OutDataTypeStr=boolean
  Relational Operator : RelationalOperator  Operator=<  OutDataTypeStr=boolean  RndMeth=Nearest
  Scope : Scope
  Subtract : Sum  Inputs=+-
  Switch : Switch  Criteria=u2 > Threshold
  Switch1 : Switch  Criteria=u2 > Threshold
  Enable : Outport
  wires:
  Compare To Zero/1 -> Logical Operator1/2
  Relational Operator/1 -> Logical Operator1/1
  Switch/1 -> Switch1/3
  Subtract/1 -> Relational Operator/1
  Digital Clock/1 -> Subtract/1
  Decision Time/1 -> Subtract/2, Compare To Zero/1
  Constant2/1 -> Switch1/1
  Constant3/1 -> Relational Operator/2
  Logical Operator1/1 -> Switch1/2, Logical Operator/1
  Switch1/1 -> Enable/1
  Logical Operator/1 -> Fixed Update Delay/1(Flag In)
  Constant/1 -> Fixed Update Delay/2(Delay), Exponential Delay/1(beta)
  Detect Increase/1 -> Switch/1, Scope/1
  Fixed Update Delay/1(Flag Out) -> Detect Increase/1
  Exponential Delay/1(Enable) -> Switch/3
  Constant1/1 -> Switch/2
